simulink model "lfm"  (R2023b)
settings: Solver=FixedStepAuto  StartTime=0.0  StopTime=10.0  FixedStep=5.3333333333333331e-09  RelTol=1e-3
undefined symbols (not defined in the file): jsin
libraries: hdlsllib x2
settings Model: Creator=mori  LastModifiedBy=mori
settings DataIOCC: SaveOutput=off  SaveTime=off

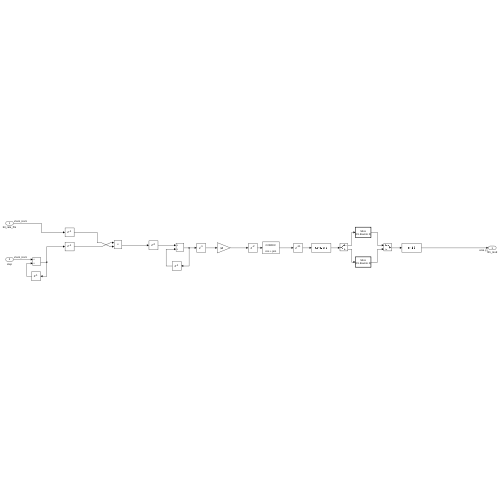
[thumbnail: Simulink's stored preview of the top-level diagram]
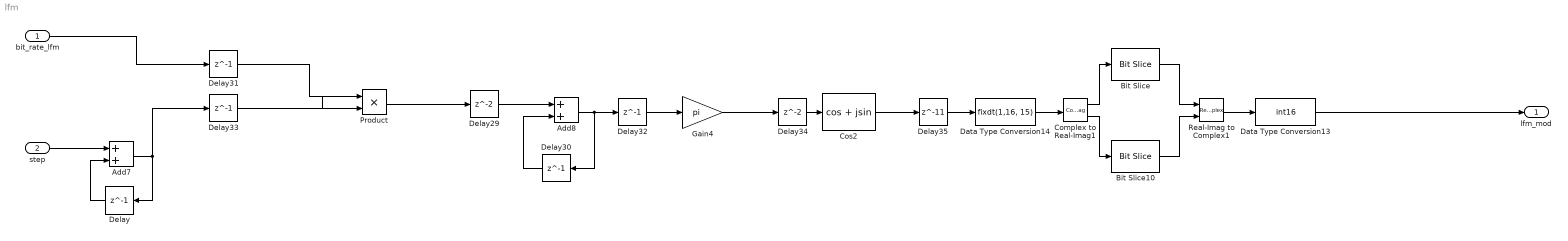
== system lfm ==
  bit_rate_lfm : Inport  OutDataTypeStr=fixdt(1,24,23)  PortDimensions=1  SampleTime=[5.3333333333333331e-09,0]
  step : Inport  Port=2  OutDataTypeStr=fixdt(1,24,23)  PortDimensions=1  SampleTime=[5.3333333333333331e-09,0]
  Add7 : Sum  OutDataTypeStr=fixdt(1,24,23)  AccumDataTypeStr=fixdt(1,24,23)
  Add8 : Sum  OutDataTypeStr=fixdt(1, 24, 23)
  Bit Slice : hdlsllib/Logic and Bit Operations/Bit Slice  lidx=15  ridx=0
  Bit Slice10 : hdlsllib/Logic and Bit Operations/Bit Slice  lidx=15  ridx=0
  Complex to Real-Imag1 : ComplexToRealImag
  Cos2 : Trigonometry  Operator=cos + jsin  ApproximationMethod=CORDIC
  Data Type Conversion13 : DataTypeConversion  OutDataTypeStr=int16  SaturateOnIntegerOverflow=off  RndMeth=Floor
  Data Type Conversion14 : DataTypeConversion  OutDataTypeStr=fixdt(1,16, 15)  RndMeth=Nearest
  Delay : Delay  DelayLength=1
  Delay29 : Delay
  Delay30 : Delay  DelayLength=1
  Delay31 : Delay  DelayLength=1  SampleTime=1/187.5e6
  Delay32 : Delay  DelayLength=1
  Delay33 : Delay  DelayLength=1  SampleTime=1/187.5e6
  Delay34 : Delay
  Delay35 : Delay  DelayLength=11
  Gain4 : Gain  Gain=pi  OutDataTypeStr=fixdt(1,24,20)
  Product : Product  OutDataTypeStr=Inherit: Same as first input
  Real-Imag to Complex1 : RealImagToComplex
  lfm_mod : Outport  OutDataTypeStr=int16  PortDimensions=1  SampleTime=[5.3333333333333331e-09,0]
      settings: SignalType=complex
  wires:
  Delay31/1 -> Product/2
  Data Type Conversion14/1 -> Complex to Real-Imag1/1
  Product/1 -> Delay29/1
  Gain4/1 -> Delay34/1
  Add8/1 -> Delay30/1, Delay32/1
  Bit Slice10/1 -> Real-Imag to Complex1/2
  Bit Slice/1 -> Real-Imag to Complex1/1
  Delay33/1 -> Product/1
  Delay32/1 -> Gain4/1
  Add7/1 -> Delay/1, Delay33/1
  Cos2/1 -> Delay35/1
  Delay30/1 -> Add8/2
  Delay34/1 -> Cos2/1
  Complex to Real-Imag1/2 -> Bit Slice10/1
  Delay/1 -> Add7/2
  Real-Imag to Complex1/1 -> Data Type Conversion13/1
  Delay35/1 -> Data Type Conversion14/1
  Complex to Real-Imag1/1 -> Bit Slice/1
  bit_rate_lfm/1 -> Delay31/1
  Data Type Conversion13/1 -> lfm_mod/1
  step/1 -> Add7/1
  Delay29/1 -> Add8/1
